simulink model "MSA_IS_dyn"  (Simulink 7.8)
settings: Solver=ode4  StartTime=0.0  StopTime=time_span-1  FixedStep=samp_time  RelTol=1e-3
undefined symbols (not defined in the file or in its folder): IC, outstr, samp_time
settings Model: Creator=danai  LastModifiedBy=TheQuarry
settings SolverCC: MaxConsecutiveMinStep=dt
settings GRTTargetCC: CombineOutputUpdateFcns=on

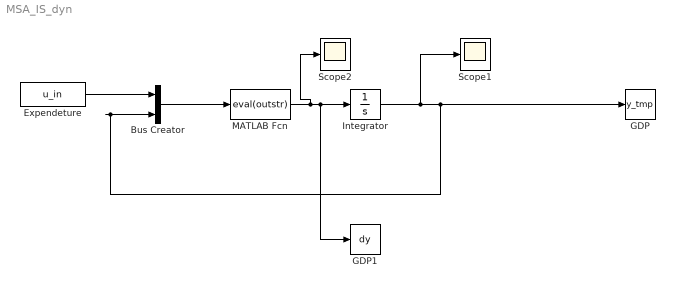
== system MSA_IS_dyn ==
  Bus Creator : BusCreator  Inputs=2
  Expendeture : FromWorkspace  VariableName=u_in  SampleTime=samp_time
  GDP : ToWorkspace  VariableName=y_tmp  SampleTime=-1  SaveFormat=Array
  GDP1 : ToWorkspace  VariableName=dy  SampleTime=-1  SaveFormat=Array
  Integrator : Integrator  InitialCondition=IC(2)
  MATLAB Fcn : MATLABFcn  MATLABFcn=eval(outstr)
  Scope1 : Scope
  Scope2 : Scope
  wires:
  Expendeture/1 -> Bus Creator/1
  Bus Creator/1 -> MATLAB Fcn/1
  MATLAB Fcn/1 -> Scope2/1, Integrator/1, GDP1/1
  Integrator/1 -> Scope1/1, Bus Creator/2, GDP/1
